simulink model "MomentCartCBAgent"  (Simulink 7.1)
settings: Solver=ode45  SolverMode=SingleTasking  StartTime=0.0  StopTime=10.0  RelTol=1e-3  AbsTol=1e-6
settings Model: Creator=The MathWorks Inc.  LastModifiedBy=suarezjl  ExtModeTrigMode=oneshot  ExtModeArmWhenConnect=off  ExtModeAutoUpdateStatusClock=off
settings DataIOCC: LimitDataPoints=off  SignalLoggingName=logsOut
settings OptimizationCC: BooleanDataType=off  InlineInvariantSignals=on
settings DebuggingCC: SaveWithParameterizedLinksMsg=none  CheckExecutionContextPreStartOutputMsg=on  CheckExecutionContextRuntimeOutputMsg=on  SignalResolutionControl=TryResolveAllWithWarning  SolverPrmCheckMsg=none  MultiTaskDSMMsg=warning  MultiTaskCondExecSysMsg=none  IntegerOverflowMsg=none  StrictBusMsg=None
settings HardwareCC: TargetUnknown=on
settings ModelReferenceCC: UpdateModelReferenceTargets=IfOutOfDate
settings RTWCC: IncludeERTFirstTime=on
settings GRTTargetCC: TargetFcnLib=ansi_tfl_tmw.mat

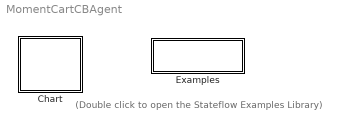
== system MomentCartCBAgent ==
  note: (Double click to open the
      | Stateflow Examples Library)
  Chart : Stateflow chart
  Examples : Subsystem
      settings: OpenFcn=sf('Private','sf_examples')
      mask Display: disp('Examples')

== system MomentCartCBAgent/Examples ==

== stateflow chart Chart ==
  state Initialize
    Aquateen\ControlBasisModuleMC\HP3JCAgent\HP3JC.connect_Initialize()
    Aquateen\ControlBasisModuleMC\HP3JCAgent\HP3JC.servo_ServoOn()
    Aquateen\ControlBasisModuleMC\HP3JCAgent\HP3JC.job_SelectJob()
    Aquateen\ControlBasisModuleMC\HP3JCAgent\HP3JC.job_StartJob()
    Aquateen\ControlBasisModuleMC\ForceSensor\StateMachine.LoadSM()
    Aquateen\ControlBasisModuleMC\ForceSensor\StateMachine.Start()
    Aquateen\ControlBasisModuleMC\HP3JCAgent\HP3JC.read_CurrentPosition()
    Aquateen\ControlBasisModuleMC\MomentCartCB\MomentCartCB.Initialize()
  state ReadPosition
    Aquateen\ControlBasisModuleMC\HP3JCAgent\HP3JC.read_CurrentPosition()
    Aquateen\ControlBasisModuleMC\MomentCartCB\MomentCartCB.ComputeControlBasis()
    Aquateen\ControlBasisModuleMC\HP3JCAgent\HP3JC.move_JointAngles()
    Aquateen\ControlBasisModuleMC\HP3JCAgent\HP3JC.move_LinearMotion()
    Aquateen\ControlBasisModuleMC\MomentCartCB\StateMachine.Wait(200)
  state Stop
    Aquateen\ControlBasisModuleMC\ForceSensor\StateMachine.Stop()
    Aquateen\ControlBasisModuleMC\HP3JCAgent\HP3JC.job_SelectJob()
    Aquateen\ControlBasisModuleMC\HP3JCAgent\HP3JC.job_StartJob()
  state \Stop
    Aquateen\ControlBasisModuleMC\ForceSensor\StateMachine.Wait(100)
  (default) -> Initialize : Start
  Initialize -> ReadPosition : Always
  ReadPosition -> ReadPosition [order 1] : Default
  ReadPosition -> \Stop [order 3] : Signal="Stop"
  ReadPosition -> Stop [order 2] : Signal="Clear"
